simulink model "CF009A_GmOvrlStMgr"  (R2013b)
settings: Solver=FixedStepDiscrete  SolverMode=SingleTasking  StartTime=0.0  StopTime=1  FixedStep=0.002  RelTol=1e-3
values from neighbouring files (symbols this model uses):
  APASTACTV_CNT_U08 = DataDict.Constant    [CF009A_GmOvrlStMgr_DataDict.m]
  APASTCTRLAVL_CNT_U08 = DataDict.Constant    [CF009A_GmOvrlStMgr_DataDict.m]
  ARCHGLBPRM_2MILLISEC_SEC_F32 = DataDict.Constant    [CF009A_GmOvrlStMgr_DataDict.m]
  GmOvrlStMgrApaHwTqThd = DataDict.Calibration    [CF009A_GmOvrlStMgr_DataDict.m]
  GmOvrlStMgrApaHwTqTiThd = DataDict.Calibration    [CF009A_GmOvrlStMgr_DataDict.m]
  GmOvrlStMgrApaMfgEna = DataDict.Calibration    [CF009A_GmOvrlStMgr_DataDict.m]
  GmOvrlStMgrEscMfgEna = DataDict.Calibration    [CF009A_GmOvrlStMgr_DataDict.m]
  GmOvrlStMgrHaptcAmp = DataDict.Calibration    [CF009A_GmOvrlStMgr_DataDict.m]
  GmOvrlStMgrHaptcDurn = DataDict.Calibration    [CF009A_GmOvrlStMgr_DataDict.m]
  GmOvrlStMgrHaptcFrq = DataDict.Calibration    [CF009A_GmOvrlStMgr_DataDict.m]
  GmOvrlStMgrHaptcReactnTi = DataDict.Calibration    [CF009A_GmOvrlStMgr_DataDict.m]
  GmOvrlStMgrHaptcReqTiThd = DataDict.Calibration    [CF009A_GmOvrlStMgr_DataDict.m]
  GmOvrlStMgrHwAgTarLimr = DataDict.Calibration    [CF009A_GmOvrlStMgr_DataDict.m]
  GmOvrlStMgrLkaHwTqThd1 = DataDict.Calibration    [CF009A_GmOvrlStMgr_DataDict.m]
  GmOvrlStMgrLkaHwTqThd2 = DataDict.Calibration    [CF009A_GmOvrlStMgr_DataDict.m]
  GmOvrlStMgrLkaHwTqTiThd1 = DataDict.Calibration    [CF009A_GmOvrlStMgr_DataDict.m]
  GmOvrlStMgrLkaHwTqTiThd2 = DataDict.Calibration    [CF009A_GmOvrlStMgr_DataDict.m]
  GmOvrlStMgrLkaMfgEna = DataDict.Calibration    [CF009A_GmOvrlStMgr_DataDict.m]
  GmOvrlStMgrLoaMtgtnHaptcFbOffTi = DataDict.Calibration    [CF009A_GmOvrlStMgr_DataDict.m]
  GmOvrlStMgrLoaMtgtnHaptcFbOnTi = DataDict.Calibration    [CF009A_GmOvrlStMgr_DataDict.m]
  GmOvrlStMgrLoaMtgtnHaptcFbStrtOnTi = DataDict.Calibration    [CF009A_GmOvrlStMgr_DataDict.m]
  GmOvrlStMgrLoaMtgtnHaptcFbTqMax = DataDict.Calibration    [CF009A_GmOvrlStMgr_DataDict.m]
  GmOvrlStMgrLoaMtgtnHaptcFbTqMin = DataDict.Calibration    [CF009A_GmOvrlStMgr_DataDict.m]
  GmOvrlStMgrLoaMtgtnHaptcFbVehSpdMax = DataDict.Calibration    [CF009A_GmOvrlStMgr_DataDict.m]
  GmOvrlStMgrLoaMtgtnHaptcFbVehSpdMin = DataDict.Calibration    [CF009A_GmOvrlStMgr_DataDict.m]
  GmOvrlStMgrLoaMtgtnHaptcFrq = DataDict.Calibration    [CF009A_GmOvrlStMgr_DataDict.m]
  GmOvrlStMgrLoaMtgtnStrtHaptcAmp = DataDict.Calibration    [CF009A_GmOvrlStMgr_DataDict.m]
  GmOvrlStMgrLoaStIgnCntrThd = DataDict.Calibration    [CF009A_GmOvrlStMgr_DataDict.m]
  GmOvrlStMgrShiftLvrTiThd = DataDict.Calibration    [CF009A_GmOvrlStMgr_DataDict.m]
  GmOvrlStMgrStandStillThd = DataDict.Calibration    [CF009A_GmOvrlStMgr_DataDict.m]
  GmOvrlStMgrStandStillTiThd = DataDict.Calibration    [CF009A_GmOvrlStMgr_DataDict.m]
  HAPTCSTACTV_CNT_U08 = DataDict.Constant    [CF009A_GmOvrlStMgr_DataDict.m]
  HAPTCSTWAIT_CNT_U08 = DataDict.Constant    [CF009A_GmOvrlStMgr_DataDict.m]
  HWOSCNFRQMIN_HZ_F32 = DataDict.Constant    [CF009A_GmOvrlStMgr_DataDict.m]
  LKAFLTCNTRTHD_CNT_U08 = DataDict.Constant    [CF009A_GmOvrlStMgr_DataDict.m]
  LKAFLTTMRTHD_MILLISEC_U32 = DataDict.Constant    [CF009A_GmOvrlStMgr_DataDict.m]
  LKASTPRMNTFAILD_CNT_U08 = DataDict.Constant    [CF009A_GmOvrlStMgr_DataDict.m]
  LoaMtgtnThdExcdd = DataDict.NTC    [CF009A_GmOvrlStMgr_DataDict.m]
  MILLISECTO100MICROSECCNVN_CNT_U32 = DataDict.Constant    [CF009A_GmOvrlStMgr_DataDict.m]
  NODEBSTEP_CNT_U16 = DataDict.Constant    [CF009A_GmOvrlStMgr_DataDict.m]
undefined symbols (not defined in the file or in its folder): LoaSt1, NtcSts1, NVM_RequestResultType, SysSt1
libraries: simulink x13, Fil x6, NxtrNvM x4, NxtrLim x4, NxtrAbslt x3, NxtrSign x2, FixdToFloat x1, FloatToFixd x1, LnrIntrpn x1
(part 5 of 8)

== system CF009A_GmOvrlStMgr/GmOvrlStMgr/GmOvrlStMgrPer1/ApaIntv/Timer for ApaIntv/If Action Subsystem2 ==
  Action Port : ActionPort  ActionType=elseif
  CopyRight2 : Subsystem  Description=|  mask(Copyright Information){none=on}
      | Copyright info block.                                               
      |                                                                     
      | Place copyright information at the top of every subsystem in design.
      mask prompts: none "No parameters"
      mask help: Place copyright information at the top of every subsystem in design.
      mask Display:
      | NxtrConf = 'Nexteer Confidential';
      | 
      | sys = bdroot; %handle for the current model ("system")
      | first = get_param(sys,'Created');
      | first = first(end-3:end);  %year is last four digits
      | 
      | last = get_param(sys,'LastModifiedDate');
      | if isempty(last)
      |     last = datestr(now,'yyyy');
      | else
      |     last = last(end-3:end);
      | end
      | 
      | if strcmp(first,last)
      |     fprintf('%s -- Copyright %s Nexteer',NxtrConf,first)
      | else
      |     fprintf('%s -- %s%s- %s Nexteer',NxtrConf,char(169),first,last)
      | end
  Data Store Read : DataStoreRead  DataStoreName=PrevApaIntvRefTi
  GetTiSpan100MicroSec32bit1 : Subsystem
  Out1 : Outport
  wires:
  GetTiSpan100MicroSec32bit1/1(TiSpan) -> Out1/1
  Data Store Read/1 -> GetTiSpan100MicroSec32bit1/1(RefTmr)

== system CF009A_GmOvrlStMgr/GmOvrlStMgr/GmOvrlStMgrPer1/HaptcStTransActvToWaitFlg/ElpseTi/CopyRight2 ==

== system CF009A_GmOvrlStMgr/GmOvrlStMgr/GmOvrlStMgrPer1/HaptcStTransActvToWaitFlg/ElpseTi/GetTiSpan100MicroSec32bit ==
  note: Subtract original reference time
  note: seconds
  note: microseconds
  note: counts
  note: Wrap-to-zero
  note: 1 count = 100 uSec
  note: Get current system time
  note: GetTiSpan100MicroSec32bit
  note: Created Aug 18, 2015
      | Modified Oct 21, 2015
      | Modified Oct 30, 2015
      | Kevin Derry
  RefTmr : Inport
  CopyRight2 : Subsystem  Description=|  mask(Copyright Information){none=on}
      | Copyright info block.                                               
      |                                                                     
      | Place copyright information at the top of every subsystem in design.
      mask prompts: none "No parameters"
      mask help: Place copyright information at the top of every subsystem in design.
      mask Display:
      | NxtrConf = 'Nexteer Confidential';
      | 
      | sys = bdroot; %handle for the current model ("system")
      | first = get_param(sys,'Created');
      | if(isempty(first))
      |     first = datestr(now,'yyyy');
      | else
      |     first = first(end-3:end);  %year is last four digits
      | end
      | 
      | last = get_param(sys,'LastModifiedDate');
      | if isempty(last)
      |     last = datestr(now,'yyyy');
      | else
      |     last = last(end-3:end);
      | end
      | 
      | if strcmp(first,last)
      |     fprintf('%s -- Copyright %s Nexteer',NxtrConf,first)
      | else
      |     fprintf('%s -- %s%s- %s Nexteer',NxtrConf,char(169),first,last)
      | end
  Count per uSec : Constant  Value=0.01
  Data Store Read1 : DataStoreRead  DataStoreName=SimnTi
  Data Type Conversion2 : DataTypeConversion  OutDataTypeStr=uint32
  Divide1 : Product  Inputs=**
  Divide2 : Product  Inputs=*/
  If : If  NumInputs=2  IfExpression=u1 >= u2
  Max Counts : Constant  Value=2^32-1
  Merge : Merge
  No wrapping : Subsystem  TreatAsAtomicUnit=on
  Product2 : Product
  Product3 : Product
  Rounding : Rounding
  Subtract3 : Sum  Inputs=+-
  Wrapping : Subsystem  TreatAsAtomicUnit=on
  uSec per Sec : Constant  Value=1000000
  TiSpan : Outport
  wires:
  Wrapping/1(Out1) -> Merge/2
  No wrapping/1(Out1) -> Merge/1
  If/2 -> Wrapping/Action
  If/1 -> No wrapping/Action
  Product3/1 -> Subtract3/2
  Subtract3/1 -> Data Type Conversion2/1
  Rounding/1 -> Product3/1
  Divide2/1 -> Rounding/1
  Max Counts/1 -> Divide2/2, Product3/2
  Divide1/1 -> Divide2/1, Subtract3/1
  Product2/1 -> Divide1/1
  Data Store Read1/1 -> Product2/1
  Count per uSec/1 -> Divide1/2
  uSec per Sec/1 -> Product2/2
  Merge/1 -> TiSpan/1
  RefTmr/1 -> If/2, No wrapping/2(ref), Wrapping/2(ref)
  Data Type Conversion2/1 -> If/1, No wrapping/1(new), Wrapping/1(new)

== system CF009A_GmOvrlStMgr/GmOvrlStMgr/GmOvrlStMgrPer1/HaptcStTransActvToWaitFlg/ElpseTi/Set False Subsystem ==
  Action Port : ActionPort  ActionType=else
  Constant1 : Constant  RequirementInfo={} %GIDa_7a5b8ee3_9c22_45c3_98e2_7098368aea92  Value=false  OutDataTypeStr=boolean
      settings: AttributesFormatString=%<OutDataTypeStr>
  CopyRight2 : Subsystem  Description=|  mask(Copyright Information){none=on}
      | Copyright info block.                                               
      |                                                                     
      | Place copyright information at the top of every subsystem in design.
      mask prompts: none "No parameters"
      mask help: Place copyright information at the top of every subsystem in design.
      mask Display:
      | NxtrConf = 'Nexteer Confidential';
      | 
      | sys = bdroot; %handle for the current model ("system")
      | first = get_param(sys,'Created');
      | first = first(end-3:end);  %year is last four digits
      | 
      | last = get_param(sys,'LastModifiedDate');
      | if isempty(last)
      |     last = datestr(now,'yyyy');
      | else
      |     last = last(end-3:end);
      | end
      | 
      | if strcmp(first,last)
      |     fprintf('%s -- Copyright %s Nexteer',NxtrConf,first)
      | else
      |     fprintf('%s -- %s%s- %s Nexteer',NxtrConf,char(169),first,last)
      | end
  Out1 : Outport
  wires:
  Constant1/1 -> Out1/1

== system CF009A_GmOvrlStMgr/GmOvrlStMgr/GmOvrlStMgrPer1/HaptcStTransActvToWaitFlg/ElpseTi/Set True Subsystem ==
  Action Port : ActionPort  ActionType=then
  Constant13 : Constant  RequirementInfo={} %GIDa_d2a44b6e_d583_493a_9335_9403f2dad45d  Value=true  OutDataTypeStr=boolean
      settings: AttributesFormatString=%<OutDataTypeStr>
  CopyRight2 : Subsystem  Description=|  mask(Copyright Information){none=on}
      | Copyright info block.                                               
      |                                                                     
      | Place copyright information at the top of every subsystem in design.
      mask prompts: none "No parameters"
      mask help: Place copyright information at the top of every subsystem in design.
      mask Display:
      | NxtrConf = 'Nexteer Confidential';
      | 
      | sys = bdroot; %handle for the current model ("system")
      | first = get_param(sys,'Created');
      | first = first(end-3:end);  %year is last four digits
      | 
      | last = get_param(sys,'LastModifiedDate');
      | if isempty(last)
      |     last = datestr(now,'yyyy');
      | else
      |     last = last(end-3:end);
      | end
      | 
      | if strcmp(first,last)
      |     fprintf('%s -- Copyright %s Nexteer',NxtrConf,first)
      | else
      |     fprintf('%s -- %s%s- %s Nexteer',NxtrConf,char(169),first,last)
      | end
  Out1 : Outport
  wires:
  Constant13/1 -> Out1/1

== system CF009A_GmOvrlStMgr/GmOvrlStMgr/GmOvrlStMgrPer1/HaptcStTransActvToWaitFlg/RefTi/CopyRight2 ==

== system CF009A_GmOvrlStMgr/GmOvrlStMgr/GmOvrlStMgrPer1/HaptcStTransActvToWaitFlg/RefTi/GetRefTmr100MicroSec32bit ==
  note: 1 count = 100 uSec
  note: seconds
  note: microseconds
  note: counts
  note: Wrap-to-zero
  note: GetRefTmr100MicroSec32bit
  note: Created Aug 18, 2015
      | Modified Oct 21, 2015
      | Modified Oct 30, 2015
      | Kevin Derry
  CopyRight2 : Subsystem  Description=|  mask(Copyright Information){none=on}
      | Copyright info block.                                               
      |                                                                     
      | Place copyright information at the top of every subsystem in design.
      mask prompts: none "No parameters"
      mask help: Place copyright information at the top of every subsystem in design.
      mask Display:
      | NxtrConf = 'Nexteer Confidential';
      | 
      | sys = bdroot; %handle for the current model ("system")
      | first = get_param(sys,'Created');
      | if(isempty(first))
      |     first = datestr(now,'yyyy');
      | else
      |     first = first(end-3:end);  %year is last four digits
      | end
      | 
      | last = get_param(sys,'LastModifiedDate');
      | if isempty(last)
      |     last = datestr(now,'yyyy');
      | else
      |     last = last(end-3:end);
      | end
      | 
      | if strcmp(first,last)
      |     fprintf('%s -- Copyright %s Nexteer',NxtrConf,first)
      | else
      |     fprintf('%s -- %s%s- %s Nexteer',NxtrConf,char(169),first,last)
      | end
  Count per uSec : Constant  Value=0.01
  Data Store Read1 : DataStoreRead  DataStoreName=SimnTi
  Data Type Conversion1 : DataTypeConversion  OutDataTypeStr=uint32
  Divide1 : Product  Inputs=**
  Divide2 : Product  Inputs=*/
  Max Counts : Constant  Value=2^32-1
  Product1 : Product
  Product2 : Product
  Rounding : Rounding
  Subtract1 : Sum  Inputs=+-
  uSec per Sec : Constant  Value=1000000
  RefTmr : Outport
  wires:
  Product2/1 -> Subtract1/2
  Subtract1/1 -> Data Type Conversion1/1
  Rounding/1 -> Product2/1
  Divide2/1 -> Rounding/1
  Max Counts/1 -> Divide2/2, Product2/2
  Divide1/1 -> Divide2/1, Subtract1/1
  Product1/1 -> Divide1/1
  Count per uSec/1 -> Divide1/2
  uSec per Sec/1 -> Product1/2
  Data Type Conversion1/1 -> RefTmr/1
  Data Store Read1/1 -> Product1/1

== system CF009A_GmOvrlStMgr/GmOvrlStMgr/GmOvrlStMgrPer1/HwAgServo/If Action Subsystem/ApaStatusActive ==
  note: Code uses magic number
  Action Port : ActionPort  ActionType=then
  Constant : Constant  Value=false
  Constant1 : Constant  Value=0  OutDataTypeStr=single
  CopyRight2 : Subsystem  Description=|  mask(Copyright Information){none=on}
      | Copyright info block.                                               
      |                                                                     
      | Place copyright information at the top of every subsystem in design.
      mask prompts: none "No parameters"
      mask help: Place copyright information at the top of every subsystem in design.
      mask Display:
      | NxtrConf = 'Nexteer Confidential';
      | 
      | sys = bdroot; %handle for the current model ("system")
      | first = get_param(sys,'Created');
      | if(isempty(first))
      |     first = datestr(now,'yyyy');
      | else
      |     first = first(end-3:end);  %year is last four digits
      | end
      | 
      | last = get_param(sys,'LastModifiedDate');
      | if isempty(last)
      |     last = datestr(now,'yyyy');
      | else
      |     last = last(end-3:end);
      | end
      | 
      | if strcmp(first,last)
      |     fprintf('%s -- Copyright %s Nexteer',NxtrConf,first)
      | else
      |     fprintf('%s -- %s%s- %s Nexteer',NxtrConf,char(169),first,last)
      | end
  HwAgServoEna : Outport
  HwAgServoCmd : Outport  Port=2
  wires:
  Constant/1 -> HwAgServoEna/1
  Constant1/1 -> HwAgServoCmd/1

== system CF009A_GmOvrlStMgr/GmOvrlStMgr/GmOvrlStMgrPer1/HwAgServo/If Action Subsystem/ApaStatusNotActive ==
  HwAgTraj : Inport
  Action Port : ActionPort  ActionType=else
  Constant : Constant  Value=true
  CopyRight2 : Subsystem  Description=|  mask(Copyright Information){none=on}
      | Copyright info block.                                               
      |                                                                     
      | Place copyright information at the top of every subsystem in design.
      mask prompts: none "No parameters"
      mask help: Place copyright information at the top of every subsystem in design.
      mask Display:
      | NxtrConf = 'Nexteer Confidential';
      | 
      | sys = bdroot; %handle for the current model ("system")
      | first = get_param(sys,'Created');
      | if(isempty(first))
      |     first = datestr(now,'yyyy');
      | else
      |     first = first(end-3:end);  %year is last four digits
      | end
      | 
      | last = get_param(sys,'LastModifiedDate');
      | if isempty(last)
      |     last = datestr(now,'yyyy');
      | else
      |     last = last(end-3:end);
      | end
      | 
      | if strcmp(first,last)
      |     fprintf('%s -- Copyright %s Nexteer',NxtrConf,first)
      | else
      |     fprintf('%s -- %s%s- %s Nexteer',NxtrConf,char(169),first,last)
      | end
  HwAgServoCmd : Outport
  HwAgServoEna : Outport  Port=2
  wires:
  Constant/1 -> HwAgServoEna/1
  HwAgTraj/1 -> HwAgServoCmd/1

== system CF009A_GmOvrlStMgr/GmOvrlStMgr/GmOvrlStMgrPer1/HwAgServo/If Action Subsystem/CopyRight2 ==

== system CF009A_GmOvrlStMgr/GmOvrlStMgr/GmOvrlStMgrPer1/HwAgServo/If Action Subsystem1/ApaStatusActive ==
  HwAgTarLimd : Inport
  Action Port : ActionPort  ActionType=then
  Constant : Constant  Value=true
  CopyRight2 : Subsystem  Description=|  mask(Copyright Information){none=on}
      | Copyright info block.                                               
      |                                                                     
      | Place copyright information at the top of every subsystem in design.
      mask prompts: none "No parameters"
      mask help: Place copyright information at the top of every subsystem in design.
      mask Display:
      | NxtrConf = 'Nexteer Confidential';
      | 
      | sys = bdroot; %handle for the current model ("system")
      | first = get_param(sys,'Created');
      | if(isempty(first))
      |     first = datestr(now,'yyyy');
      | else
      |     first = first(end-3:end);  %year is last four digits
      | end
      | 
      | last = get_param(sys,'LastModifiedDate');
      | if isempty(last)
      |     last = datestr(now,'yyyy');
      | else
      |     last = last(end-3:end);
      | end
      | 
      | if strcmp(first,last)
      |     fprintf('%s -- Copyright %s Nexteer',NxtrConf,first)
      | else
      |     fprintf('%s -- %s%s- %s Nexteer',NxtrConf,char(169),first,last)
      | end
  HwAgServoCmd : Outport
  HwAgServoEna : Outport  Port=2
  wires:
  Constant/1 -> HwAgServoEna/1
  HwAgTarLimd/1 -> HwAgServoCmd/1

== system CF009A_GmOvrlStMgr/GmOvrlStMgr/GmOvrlStMgrPer1/HwAgServo/If Action Subsystem1/ApaStatusNotActive ==
  note: Code uses magic number
  Action Port : ActionPort  ActionType=else
  Constant1 : Constant  Value=false
  Constant2 : Constant  Value=0  OutDataTypeStr=single
  CopyRight2 : Subsystem  Description=|  mask(Copyright Information){none=on}
      | Copyright info block.                                               
      |                                                                     
      | Place copyright information at the top of every subsystem in design.
      mask prompts: none "No parameters"
      mask help: Place copyright information at the top of every subsystem in design.
      mask Display:
      | NxtrConf = 'Nexteer Confidential';
      | 
      | sys = bdroot; %handle for the current model ("system")
      | first = get_param(sys,'Created');
      | if(isempty(first))
      |     first = datestr(now,'yyyy');
      | else
      |     first = first(end-3:end);  %year is last four digits
      | end
      | 
      | last = get_param(sys,'LastModifiedDate');
      | if isempty(last)
      |     last = datestr(now,'yyyy');
      | else
      |     last = last(end-3:end);
      | end
      | 
      | if strcmp(first,last)
      |     fprintf('%s -- Copyright %s Nexteer',NxtrConf,first)
      | else
      |     fprintf('%s -- %s%s- %s Nexteer',NxtrConf,char(169),first,last)
      | end
  HwAgServoEna : Outport
  HwAgServoCmd : Outport  Port=2
  wires:
  Constant1/1 -> HwAgServoEna/1
  Constant2/1 -> HwAgServoCmd/1

== system CF009A_GmOvrlStMgr/GmOvrlStMgr/GmOvrlStMgrPer1/HwAgServo/If Action Subsystem1/CopyRight2 ==

== system CF009A_GmOvrlStMgr/GmOvrlStMgr/GmOvrlStMgrPer1/Inct_IgnCntr_Once/IgnCntr/CopyRight2 ==

== system CF009A_GmOvrlStMgr/GmOvrlStMgr/GmOvrlStMgrPer1/LKAIntv/HwTqLkaTqSignEqu/CopyRight2 ==

== system CF009A_GmOvrlStMgr/GmOvrlStMgr/GmOvrlStMgrPer1/LKAIntv/HwTqLkaTqSignEqu/GetRefTmr100MicroSec32bit ==
  note: Created Aug 18, 2015
      | Modified Oct 21, 2015
      | Modified Oct 30, 2015
      | Kevin Derry
  note: GetRefTmr100MicroSec32bit
  note: Wrap-to-zero
  note: counts
  note: microseconds
  note: seconds
  note: 1 count = 100 uSec
  CopyRight2 : Subsystem  Description=|  mask(Copyright Information){none=on}
      | Copyright info block.                                               
      |                                                                     
      | Place copyright information at the top of every subsystem in design.
      mask prompts: none "No parameters"
      mask help: Place copyright information at the top of every subsystem in design.
      mask Display:
      | NxtrConf = 'Nexteer Confidential';
      | 
      | sys = bdroot; %handle for the current model ("system")
      | first = get_param(sys,'Created');
      | if(isempty(first))
      |     first = datestr(now,'yyyy');
      | else
      |     first = first(end-3:end);  %year is last four digits
      | end
      | 
      | last = get_param(sys,'LastModifiedDate');
      | if isempty(last)
      |     last = datestr(now,'yyyy');
      | else
      |     last = last(end-3:end);
      | end
      | 
      | if strcmp(first,last)
      |     fprintf('%s -- Copyright %s Nexteer',NxtrConf,first)
      | else
      |     fprintf('%s -- %s%s- %s Nexteer',NxtrConf,char(169),first,last)
      | end
  Count per uSec : Constant  Value=0.01
  Data Store Read1 : DataStoreRead  DataStoreName=SimnTi
  Data Type Conversion1 : DataTypeConversion  OutDataTypeStr=uint32
  Divide1 : Product  Inputs=**
  Divide2 : Product  Inputs=*/
  Max Counts : Constant  Value=2^32-1
  Product1 : Product
  Product2 : Product
  Rounding : Rounding
  Subtract1 : Sum  Inputs=+-
  uSec per Sec : Constant  Value=1000000
  RefTmr : Outport
  wires:
  Data Store Read1/1 -> Product1/1
  Data Type Conversion1/1 -> RefTmr/1
  uSec per Sec/1 -> Product1/2
  Count per uSec/1 -> Divide1/2
  Product1/1 -> Divide1/1
  Divide1/1 -> Subtract1/1, Divide2/1
  Max Counts/1 -> Product2/2, Divide2/2
  Divide2/1 -> Rounding/1
  Rounding/1 -> Product2/1
  Subtract1/1 -> Data Type Conversion1/1
  Product2/1 -> Subtract1/2

== system CF009A_GmOvrlStMgr/GmOvrlStMgr/GmOvrlStMgrPer1/LKAIntv/HwTqLkaTqSignEqu/GetRefTmr100MicroSec32bit_1 ==
  note: 1 count = 100 uSec
  note: seconds
  note: microseconds
  note: counts
  note: Wrap-to-zero
  note: GetRefTmr100MicroSec32bit
  note: Created Aug 18, 2015
      | Modified Oct 21, 2015
      | Modified Oct 30, 2015
      | Kevin Derry
  CopyRight2 : Subsystem  Description=|  mask(Copyright Information){none=on}
      | Copyright info block.                                               
      |                                                                     
      | Place copyright information at the top of every subsystem in design.
      mask prompts: none "No parameters"
      mask help: Place copyright information at the top of every subsystem in design.
      mask Display:
      | NxtrConf = 'Nexteer Confidential';
      | 
      | sys = bdroot; %handle for the current model ("system")
      | first = get_param(sys,'Created');
      | if(isempty(first))
      |     first = datestr(now,'yyyy');
      | else
      |     first = first(end-3:end);  %year is last four digits
      | end
      | 
      | last = get_param(sys,'LastModifiedDate');
      | if isempty(last)
      |     last = datestr(now,'yyyy');
      | else
      |     last = last(end-3:end);
      | end
      | 
      | if strcmp(first,last)
      |     fprintf('%s -- Copyright %s Nexteer',NxtrConf,first)
      | else
      |     fprintf('%s -- %s%s- %s Nexteer',NxtrConf,char(169),first,last)
      | end
  Count per uSec : Constant  Value=0.01
  Data Store Read1 : DataStoreRead  DataStoreName=SimnTi
  Data Type Conversion1 : DataTypeConversion  OutDataTypeStr=uint32
  Divide1 : Product  Inputs=**
  Divide2 : Product  Inputs=*/
  Max Counts : Constant  Value=2^32-1
  Product1 : Product
  Product2 : Product
  Rounding : Rounding
  Subtract1 : Sum  Inputs=+-
  uSec per Sec : Constant  Value=1000000
  RefTmr : Outport
  wires:
  Product2/1 -> Subtract1/2
  Subtract1/1 -> Data Type Conversion1/1
  Rounding/1 -> Product2/1
  Divide2/1 -> Rounding/1
  Max Counts/1 -> Divide2/2, Product2/2
  Divide1/1 -> Divide2/1, Subtract1/1
  Product1/1 -> Divide1/1
  Count per uSec/1 -> Divide1/2
  uSec per Sec/1 -> Product1/2
  Data Type Conversion1/1 -> RefTmr/1
  Data Store Read1/1 -> Product1/1

== system CF009A_GmOvrlStMgr/GmOvrlStMgr/GmOvrlStMgrPer1/LKAIntv/HwTqLkaTqSignNotEqu/ChkTmr1 ==
  Action Port : ActionPort  ActionType=then
  Constant : Constant  RequirementInfo={} %GIDa_31957342_5e2f_4bc5_989e_9132f947ba0e  Value=GmOvrlStMgrLkaHwTqTiThd1
  Constant1 : Constant  Value=MILLISECTO100MICROSECCNVN_CNT_U32
  CopyRight2 : Subsystem  Description=|  mask(Copyright Information){none=on}
      | Copyright info block.                                               
      |                                                                     
      | Place copyright information at the top of every subsystem in design.
      mask prompts: none "No parameters"
      mask help: Place copyright information at the top of every subsystem in design.
      mask Display:
      | NxtrConf = 'Nexteer Confidential';
      | 
      | sys = bdroot; %handle for the current model ("system")
      | first = get_param(sys,'Created');
      | if(isempty(first))
      |     first = datestr(now,'yyyy');
      | else
      |     first = first(end-3:end);  %year is last four digits
      | end
      | 
      | last = get_param(sys,'LastModifiedDate');
      | if isempty(last)
      |     last = datestr(now,'yyyy');
      | else
      |     last = last(end-3:end);
      | end
      | 
      | if strcmp(first,last)
      |     fprintf('%s -- Copyright %s Nexteer',NxtrConf,first)
      | else
      |     fprintf('%s -- %s%s- %s Nexteer',NxtrConf,char(169),first,last)
      | end
  Data Store Read : DataStoreRead  DataStoreName=LkaIntvRefTi1
  Data Store Write1 : DataStoreWrite  DataStoreName=LkaIntvRefTi2
  GetRefTmr100MicroSec32bit : Subsystem
  GetTiSpan100MicroSec32bit : Subsystem
  If1 : If  IfExpression=u1
  LKAIntvTi1Elpd : Subsystem
  LKAIntvTi1NotElpd : Subsystem
  Merge3 : Merge
  Product1 : Product
  Relational Operator : RelationalOperator  OutDataTypeStr=boolean
  Out1 : Outport
  wires:
  Merge3/1 -> Out1/1
  LKAIntvTi1NotElpd/1(Out1) -> Merge3/2
  LKAIntvTi1Elpd/1(Out1) -> Merge3/1
  If1/2 -> LKAIntvTi1NotElpd/Action
  If1/1 -> LKAIntvTi1Elpd/Action
  Constant/1 -> Product1/1
  Product1/1 -> Relational Operator/2
  Constant1/1 -> Product1/2
  Relational Operator/1 -> If1/1
  GetTiSpan100MicroSec32bit/1(TiSpan) -> Relational Operator/1
  Data Store Read/1 -> GetTiSpan100MicroSec32bit/1(RefTmr)
  GetRefTmr100MicroSec32bit/1(RefTmr) -> Data Store Write1/1

== system CF009A_GmOvrlStMgr/GmOvrlStMgr/GmOvrlStMgrPer1/LKAIntv/HwTqLkaTqSignNotEqu/ChkTmr2 ==
  Action Port : ActionPort  ActionType=elseif
  Constant : Constant  RequirementInfo={} %GIDa_932db252_e6c8_4b41_be46_d3f1492e3714  Value=GmOvrlStMgrLkaHwTqTiThd2
  Constant1 : Constant  Value=MILLISECTO100MICROSECCNVN_CNT_U32
  CopyRight2 : Subsystem  Description=|  mask(Copyright Information){none=on}
      | Copyright info block.                                               
      |                                                                     
      | Place copyright information at the top of every subsystem in design.
      mask prompts: none "No parameters"
      mask help: Place copyright information at the top of every subsystem in design.
      mask Display:
      | NxtrConf = 'Nexteer Confidential';
      | 
      | sys = bdroot; %handle for the current model ("system")
      | first = get_param(sys,'Created');
      | first = first(end-3:end);  %year is last four digits
      | 
      | last = get_param(sys,'LastModifiedDate');
      | if isempty(last)
      |     last = datestr(now,'yyyy');
      | else
      |     last = last(end-3:end);
      | end
      | 
      | if strcmp(first,last)
      |     fprintf('%s -- Copyright %s Nexteer',NxtrConf,first)
      | else
      |     fprintf('%s -- %s%s- %s Nexteer',NxtrConf,char(169),first,last)
      | end
  Data Store Read : DataStoreRead  DataStoreName=LkaIntvRefTi2
  Data Store Write9 : DataStoreWrite  DataStoreName=LkaIntvRefTi1
  GetRefTmr100MicroSec32bit : Subsystem
  GetTiSpan100MicroSec32bit : Subsystem
  If1 : If  IfExpression=u1
  LKAIntvTi2Elpd : Subsystem
  LKAIntvTi2NotElpd : Subsystem
  Merge3 : Merge
  Product1 : Product
  Relational Operator : RelationalOperator  OutDataTypeStr=boolean
  Out1 : Outport
  wires:
  Data Store Read/1 -> GetTiSpan100MicroSec32bit/1(RefTmr)
  GetTiSpan100MicroSec32bit/1(TiSpan) -> Relational Operator/1
  Relational Operator/1 -> If1/1
  Constant1/1 -> Product1/2
  Product1/1 -> Relational Operator/2
  Constant/1 -> Product1/1
  If1/1 -> LKAIntvTi2Elpd/Action
  If1/2 -> LKAIntvTi2NotElpd/Action
  LKAIntvTi2NotElpd/1(Out1) -> Merge3/2
  Merge3/1 -> Out1/1
  GetRefTmr100MicroSec32bit/1(RefTmr) -> Data Store Write9/1
  LKAIntvTi2Elpd/1(Out1) -> Merge3/1

== system CF009A_GmOvrlStMgr/GmOvrlStMgr/GmOvrlStMgrPer1/LKAIntv/HwTqLkaTqSignNotEqu/CopyRight2 ==

== system CF009A_GmOvrlStMgr/GmOvrlStMgr/GmOvrlStMgrPer1/LKAIntv/HwTqLkaTqSignNotEqu/TmrRst ==
  Action Port : ActionPort  ActionType=else
  Constant13 : Constant  RequirementInfo={} %GIDa_6df395ac_9b22_44c0_88b8_346f6118ff67  Value=false  OutDataTypeStr=boolean
      settings: AttributesFormatString=%<OutDataTypeStr>
  CopyRight2 : Subsystem  Description=|  mask(Copyright Information){none=on}
      | Copyright info block.                                               
      |                                                                     
      | Place copyright information at the top of every subsystem in design.
      mask prompts: none "No parameters"
      mask help: Place copyright information at the top of every subsystem in design.
      mask Display:
      | NxtrConf = 'Nexteer Confidential';
      | 
      | sys = bdroot; %handle for the current model ("system")
      | first = get_param(sys,'Created');
      | first = first(end-3:end);  %year is last four digits
      | 
      | last = get_param(sys,'LastModifiedDate');
      | if isempty(last)
      |     last = datestr(now,'yyyy');
      | else
      |     last = last(end-3:end);
      | end
      | 
      | if strcmp(first,last)
      |     fprintf('%s -- Copyright %s Nexteer',NxtrConf,first)
      | else
      |     fprintf('%s -- %s%s- %s Nexteer',NxtrConf,char(169),first,last)
      | end
  Data Store Write1 : DataStoreWrite  DataStoreName=LkaIntvRefTi2
  Data Store Write9 : DataStoreWrite  DataStoreName=LkaIntvRefTi1
  GetRefTmr100MicroSec32bit : Subsystem
  GetRefTmr100MicroSec32bit_1 : Subsystem
  Out1 : Outport
  wires:
  Constant13/1 -> Out1/1
  GetRefTmr100MicroSec32bit/1(RefTmr) -> Data Store Write9/1
  GetRefTmr100MicroSec32bit_1/1(RefTmr) -> Data Store Write1/1

== system CF009A_GmOvrlStMgr/GmOvrlStMgr/GmOvrlStMgrPer1/LkaCheck/ProcessInp/CopyRight2 ==

== system CF009A_GmOvrlStMgr/GmOvrlStMgr/GmOvrlStMgrPer1/LkaCheck/ProcessInp/Inct_LkaFltCntr_One ==
  Action Port : ActionPort  ActionType=then
  Constant1 : Constant  Value=LKAFLTCNTRTHD_CNT_U08
  Constant2 : Constant  Value=LKAFLTCNTRTHD_CNT_U08
  CopyRight2 : Subsystem  Description=|  mask(Copyright Information){none=on}
      | Copyright info block.                                               
      |                                                                     
      | Place copyright information at the top of every subsystem in design.
      mask prompts: none "No parameters"
      mask help: Place copyright information at the top of every subsystem in design.
      mask Display:
      | NxtrConf = 'Nexteer Confidential';
      | 
      | sys = bdroot; %handle for the current model ("system")
      | first = get_param(sys,'Created');
      | if(isempty(first))
      |     first = datestr(now,'yyyy');
      | else
      |     first = first(end-3:end);  %year is last four digits
      | end
      | 
      | last = get_param(sys,'LastModifiedDate');
      | if isempty(last)
      |     last = datestr(now,'yyyy');
      | else
      |     last = last(end-3:end);
      | end
      | 
      | if strcmp(first,last)
      |     fprintf('%s -- Copyright %s Nexteer',NxtrConf,first)
      | else
      |     fprintf('%s -- %s%s- %s Nexteer',NxtrConf,char(169),first,last)
      | end
  Data Store Read1 : DataStoreRead  DataStoreName=LkaFltCntr
  Data Store Read2 : DataStoreRead  DataStoreName=LkaFltCntr
  Data Store Write1 : DataStoreWrite  DataStoreName=LkaFltCntr
  If : If  IfExpression=u1
  Inct One : Subsystem  TreatAsAtomicUnit=on
  Merge : Merge
  Relational Operator : RelationalOperator  Operator=<  OutDataTypeStr=boolean
  Saturate At 255 : Subsystem  TreatAsAtomicUnit=on
  LkaFltCntr : Outport
  wires:
  Data Store Read1/1 -> Relational Operator/1
  Relational Operator/1 -> If/1
  If/1 -> Inct One/Action
  Data Store Read2/1 -> Inct One/1(In1)
  Inct One/1(Out1) -> Merge/1
  Merge/1 -> LkaFltCntr/1, Data Store Write1/1
  Saturate At 255/1(Out1) -> Merge/2
  If/2 -> Saturate At 255/Action
  Constant2/1 -> Saturate At 255/1(In1)
  Constant1/1 -> Relational Operator/2

== system CF009A_GmOvrlStMgr/GmOvrlStMgr/GmOvrlStMgrPer1/LkaCheck/SetDefVal/CopyRight2 ==

== system CF009A_GmOvrlStMgr/GmOvrlStMgr/GmOvrlStMgrPer1/LkaCheck/TmrElpdDetn/CopyRight2 ==

== system CF009A_GmOvrlStMgr/GmOvrlStMgr/GmOvrlStMgrPer1/LkaCheck/TmrElpdDetn/GetTiSpan100MicroSec32bit ==
  note: Subtract original reference time
  note: seconds
  note: microseconds
  note: counts
  note: Wrap-to-zero
  note: 1 count = 100 uSec
  note: Get current system time
  note: GetTiSpan100MicroSec32bit
  note: Created Aug 18, 2015
      | Modified Oct 21, 2015
      | Modified Oct 30, 2015
      | Kevin Derry
  RefTmr : Inport
  CopyRight2 : Subsystem  Description=|  mask(Copyright Information){none=on}
      | Copyright info block.                                               
      |                                                                     
      | Place copyright information at the top of every subsystem in design.
      mask prompts: none "No parameters"
      mask help: Place copyright information at the top of every subsystem in design.
      mask Display:
      | NxtrConf = 'Nexteer Confidential';
      | 
      | sys = bdroot; %handle for the current model ("system")
      | first = get_param(sys,'Created');
      | if(isempty(first))
      |     first = datestr(now,'yyyy');
      | else
      |     first = first(end-3:end);  %year is last four digits
      | end
      | 
      | last = get_param(sys,'LastModifiedDate');
      | if isempty(last)
      |     last = datestr(now,'yyyy');
      | else
      |     last = last(end-3:end);
      | end
      | 
      | if strcmp(first,last)
      |     fprintf('%s -- Copyright %s Nexteer',NxtrConf,first)
      | else
      |     fprintf('%s -- %s%s- %s Nexteer',NxtrConf,char(169),first,last)
      | end
  Count per uSec : Constant  Value=0.01
  Data Store Read1 : DataStoreRead  DataStoreName=SimnTi
  Data Type Conversion2 : DataTypeConversion  OutDataTypeStr=uint32
  Divide1 : Product  Inputs=**
  Divide2 : Product  Inputs=*/
  If : If  NumInputs=2  IfExpression=u1 >= u2
  Max Counts : Constant  Value=2^32-1
  Merge : Merge
  No wrapping : Subsystem  TreatAsAtomicUnit=on
  Product2 : Product
  Product3 : Product
  Rounding : Rounding
  Subtract3 : Sum  Inputs=+-
  Wrapping : Subsystem  TreatAsAtomicUnit=on
  uSec per Sec : Constant  Value=1000000
  TiSpan : Outport
  wires:
  Wrapping/1(Out1) -> Merge/2
  No wrapping/1(Out1) -> Merge/1
  If/2 -> Wrapping/Action
  If/1 -> No wrapping/Action
  Product3/1 -> Subtract3/2
  Subtract3/1 -> Data Type Conversion2/1
  Rounding/1 -> Product3/1
  Divide2/1 -> Rounding/1
  Max Counts/1 -> Divide2/2, Product3/2
  Divide1/1 -> Divide2/1, Subtract3/1
  Product2/1 -> Divide1/1
  Data Store Read1/1 -> Product2/1
  Count per uSec/1 -> Divide1/2
  uSec per Sec/1 -> Product2/2
  Merge/1 -> TiSpan/1
  RefTmr/1 -> If/2, No wrapping/2(ref), Wrapping/2(ref)
  Data Type Conversion2/1 -> If/1, No wrapping/1(new), Wrapping/1(new)

== system CF009A_GmOvrlStMgr/GmOvrlStMgr/GmOvrlStMgrPer1/LoaStLimdOrSwBasdMtgtn/Set_false_LoaStLimdOrSwBasdMtgtn/CopyRight2 ==

== system CF009A_GmOvrlStMgr/GmOvrlStMgr/GmOvrlStMgrPer1/LoaStLimdOrSwBasdMtgtn/Set_true_LoaStLimdOrSwBasdMtgtn/CopyRight2 ==

== system CF009A_GmOvrlStMgr/GmOvrlStMgr/GmOvrlStMgrPer1/SysStOperate/Chk_LoaSt_IgnCntr_ AtStartUp/CopyRight2 ==

== system CF009A_GmOvrlStMgr/GmOvrlStMgr/GmOvrlStMgrPer1/SysStOperate/Chk_LoaSt_IgnCntr_ AtStartUp/HaptcFbOn ==
  Action Port : ActionPort  ActionType=then
  Constant : Constant  RequirementInfo={} %GIDa_d634b896_4353_4d58_aab3_1388ff4e5a7e  Value=GmOvrlStMgrLoaMtgtnHaptcFbStrtOnTi
  Constant1 : Constant  Value=MILLISECTO100MICROSECCNVN_CNT_U32
  Constant13 : Constant  RequirementInfo={} %GIDa_262c0b0f_a1c7_4cb6_a322_56f022c443b4  Value=true  OutDataTypeStr=boolean
      settings: AttributesFormatString=%<OutDataTypeStr>
  Constant2 : Constant  RequirementInfo={} %GIDa_0e0c1627_bd48_4b73_8c17_b3e71d289e10  Value=GmOvrlStMgrLoaMtgtnStrtHaptcAmp
  Constant3 : Constant  RequirementInfo={} %GIDa_1283bd5f_c42e_4786_be01_cb33c6733a49  Value=GmOvrlStMgrLoaMtgtnHaptcFrq
  CopyRight2 : Subsystem  Description=|  mask(Copyright Information){none=on}
      | Copyright info block.                                               
      |                                                                     
      | Place copyright information at the top of every subsystem in design.
      mask prompts: none "No parameters"
      mask help: Place copyright information at the top of every subsystem in design.
      mask Display:
      | NxtrConf = 'Nexteer Confidential';
      | 
      | sys = bdroot; %handle for the current model ("system")
      | first = get_param(sys,'Created');
      | if(isempty(first))
      |     first = datestr(now,'yyyy');
      | else
      |     first = first(end-3:end);  %year is last four digits
      | end
      | 
      | last = get_param(sys,'LastModifiedDate');
      | if isempty(last)
      |     last = datestr(now,'yyyy');
      | else
      |     last = last(end-3:end);
      | end
      | 
      | if strcmp(first,last)
      |     fprintf('%s -- Copyright %s Nexteer',NxtrConf,first)
      | else
      |     fprintf('%s -- %s%s- %s Nexteer',NxtrConf,char(169),first,last)
      | end
  Data Store Read : DataStoreRead  DataStoreName=LoaMtgtnHaptcFbStrtOnRefTi
  GetTiSpan100MicroSec32bit : Subsystem
  If4 : If  IfExpression=u1  ShowElse=off
  Product1 : Product
  Relational Operator : RelationalOperator  OutDataTypeStr=boolean
  Set_True_LoaStAlreadyChk : Subsystem  TreatAsAtomicUnit=on
  HaptcFbEn : Outport
  HwOscnMotAmp : Outport  RequirementInfo={} %GIDa_da8b7ae1_79c3_4630_835c_267660e443df  Port=2
  HwOscnFrq : Outport  RequirementInfo={} %GIDa_fa4c2daf_88d1_442e_8c15_e617778cd142  Port=3
  wires:
  Constant/1 -> Product1/1
  Product1/1 -> Relational Operator/2
  Constant1/1 -> Product1/2
  If4/1 -> Set_True_LoaStAlreadyChk/Action
  Relational Operator/1 -> If4/1
  Data Store Read/1 -> GetTiSpan100MicroSec32bit/1(RefTmr)
  GetTiSpan100MicroSec32bit/1(TiSpan) -> Relational Operator/1
  Constant13/1 -> HaptcFbEn/1
  Constant3/1 -> HwOscnFrq/1
  Constant2/1 -> HwOscnMotAmp/1

== system CF009A_GmOvrlStMgr/GmOvrlStMgr/GmOvrlStMgrPer1/SysStOperate/Chk_LoaSt_IgnCntr_ AtStartUp/Set_True_LoaStAlreadyChk_HaptcFbOff ==
  Action Port : ActionPort  ActionType=else
  Constant : Constant  Value=0  OutDataTypeStr=single
  Constant1 : Constant  Value=HWOSCNFRQMIN_HZ_F32  OutDataTypeStr=single
  Constant2 : Constant  Value=true  OutDataTypeStr=boolean
      settings: AttributesFormatString=%<OutDataTypeStr>
  Constant9 : Constant  Value=false  OutDataTypeStr=boolean
      settings: AttributesFormatString=%<OutDataTypeStr>
  CopyRight2 : Subsystem  Description=|  mask(Copyright Information){none=on}
      | Copyright info block.                                               
      |                                                                     
      | Place copyright information at the top of every subsystem in design.
      mask prompts: none "No parameters"
      mask help: Place copyright information at the top of every subsystem in design.
      mask Display:
      | NxtrConf = 'Nexteer Confidential';
      | 
      | sys = bdroot; %handle for the current model ("system")
      | first = get_param(sys,'Created');
      | first = first(end-3:end);  %year is last four digits
      | 
      | last = get_param(sys,'LastModifiedDate');
      | if isempty(last)
      |     last = datestr(now,'yyyy');
      | else
      |     last = last(end-3:end);
      | end
      | 
      | if strcmp(first,last)
      |     fprintf('%s -- Copyright %s Nexteer',NxtrConf,first)
      | else
      |     fprintf('%s -- %s%s- %s Nexteer',NxtrConf,char(169),first,last)
      | end
  Data Store Write1 : DataStoreWrite  DataStoreName=LoaMtgtnHaptcFbStrtOnRefTi
  Data Store Write8 : DataStoreWrite  DataStoreName=LoaStChk
  GetRefTmr100MicroSec32bit : Subsystem
  HwOscnEna : Outport  RequirementInfo={} %GIDa_8b27570c_f12a_44bd_9f1b_a12f105bfe32
  HwOscnMotAmp : Outport  RequirementInfo={} %GIDa_9bc8c96c_d837_4e6b_9d2a_397928442c6b  Port=2
  HwOscnFrq : Outport  RequirementInfo={} %GIDa_14cb683a_9a4e_4ed2_8a6e_fb06c6026e0e  Port=3
  wires:
  GetRefTmr100MicroSec32bit/1(RefTmr) -> Data Store Write1/1
  Constant1/1 -> HwOscnFrq/1
  Constant/1 -> HwOscnMotAmp/1
  Constant9/1 -> HwOscnEna/1
  Constant2/1 -> Data Store Write8/1

== system CF009A_GmOvrlStMgr/GmOvrlStMgr/GmOvrlStMgrPer1/SysStOperate/Get_HaptcFb_After_StartUp/APAStAvl_AaptcStActv ==
  Action Port : ActionPort  ActionType=then
  Constant2 : Constant  RequirementInfo={} %GIDa_26ed30cd_65b7_497c_99c0_2c1cfdd65d5d  Value=GmOvrlStMgrHaptcAmp
  Constant3 : Constant  RequirementInfo={} %GIDa_3af3e024_021c_4d8b_9358_e76bd2cbdf8f  Value=GmOvrlStMgrHaptcFrq
  Constant9 : Constant  Value=true  OutDataTypeStr=boolean
      settings: AttributesFormatString=%<OutDataTypeStr>
  CopyRight2 : Subsystem  Description=|  mask(Copyright Information){none=on}
      | Copyright info block.                                               
      |                                                                     
      | Place copyright information at the top of every subsystem in design.
      mask prompts: none "No parameters"
      mask help: Place copyright information at the top of every subsystem in design.
      mask Display:
      | NxtrConf = 'Nexteer Confidential';
      | 
      | sys = bdroot; %handle for the current model ("system")
      | first = get_param(sys,'Created');
      | if(isempty(first))
      |     first = datestr(now,'yyyy');
      | else
      |     first = first(end-3:end);  %year is last four digits
      | end
      | 
      | last = get_param(sys,'LastModifiedDate');
      | if isempty(last)
      |     last = datestr(now,'yyyy');
      | else
      |     last = last(end-3:end);
      | end
      | 
      | if strcmp(first,last)
      |     fprintf('%s -- Copyright %s Nexteer',NxtrConf,first)
      | else
      |     fprintf('%s -- %s%s- %s Nexteer',NxtrConf,char(169),first,last)
      | end
  HwOscnEna : Outport  RequirementInfo={} %GIDa_47629f5c_8f25_4666_a146_71f8917c2095
  HwOscnMotAmp : Outport  RequirementInfo={} %GIDa_7d1b9b8e_a4d9_4512_9671_cecba50286e4  Port=2
  HwOscnFrq : Outport  RequirementInfo={} %GIDa_40ff6541_bf70_433b_bf6e_81869915c99d  Port=3
  wires:
  Constant3/1 -> HwOscnFrq/1
  Constant2/1 -> HwOscnMotAmp/1
  Constant9/1 -> HwOscnEna/1

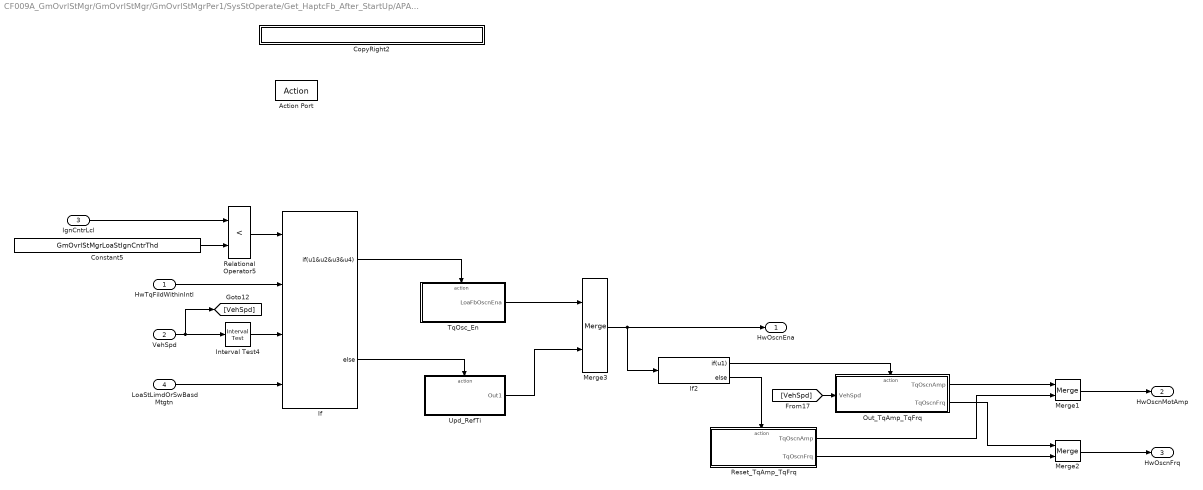
== system CF009A_GmOvrlStMgr/GmOvrlStMgr/GmOvrlStMgrPer1/SysStOperate/Get_HaptcFb_After_StartUp/APASt_NotAvl ==
  HwTqFildWithinIntl : Inport  RequirementInfo={} %GIDa_cc459f4f_ef8a_4d60_8375_9eec1001a331
  VehSpd : Inport  RequirementInfo={} %GIDa_7470b054_27ec_4b2a_a6ea_1766faf4dbc1  Port=2
  IgnCntrLcl : Inport  RequirementInfo={} %GIDa_7f00c7e6_1dc5_493c_83e8_51fe96291a10  Port=3
  LoaStLimdOrSwBasdMtgtn : Inport  RequirementInfo={} %GIDa_d7ddf5d2_779e_4bc0_a066_f8d511380f7a  Port=4
  Action Port : ActionPort  ActionType=elseif
  Constant5 : Constant  Value=GmOvrlStMgrLoaStIgnCntrThd
  CopyRight2 : Subsystem  Description=|  mask(Copyright Information){none=on}
      | Copyright info block.                                               
      |                                                                     
      | Place copyright information at the top of every subsystem in design.
      mask prompts: none "No parameters"
      mask help: Place copyright information at the top of every subsystem in design.
      mask Display:
      | NxtrConf = 'Nexteer Confidential';
      | 
      | sys = bdroot; %handle for the current model ("system")
      | first = get_param(sys,'Created');
      | if(isempty(first))
      |     first = datestr(now,'yyyy');
      | else
      |     first = first(end-3:end);  %year is last four digits
      | end
      | 
      | last = get_param(sys,'LastModifiedDate');
      | if isempty(last)
      |     last = datestr(now,'yyyy');
      | else
      |     last = last(end-3:end);
      | end
      | 
      | if strcmp(first,last)
      |     fprintf('%s -- Copyright %s Nexteer',NxtrConf,first)
      | else
      |     fprintf('%s -- %s%s- %s Nexteer',NxtrConf,char(169),first,last)
      | end
  If : If  NumInputs=4  IfExpression=u1&u2&u3&u4
  If2 : If  IfExpression=u1
  Interval Test4 : simulink/Logic and Bit Operations/Interval Test  IntervalClosedRight=on  uplimit=GmOvrlStMgrLoaMtgtnHaptcFbVehSpdMax  IntervalClosedLeft=on  lowlimit=GmOvrlStMgrLoaMtgtnHaptcFbVehSpdMin  OutDataTypeStr=boolean
  Merge1 : Merge
  Merge2 : Merge
  Merge3 : Merge
  Out_TqAmp_TqFrq : Subsystem  TreatAsAtomicUnit=on
  Relational Operator5 : RelationalOperator  Operator=<  OutDataTypeStr=boolean
  Reset_TqAmp_TqFrq : Subsystem  TreatAsAtomicUnit=on
  TqOsc_En : Subsystem  TreatAsAtomicUnit=on
  Upd_RefTi : Subsystem  TreatAsAtomicUnit=on
  HwOscnEna : Outport  RequirementInfo={} %GIDa_5788a13f_5bc7_4cac_a2cd_7377a94a3611
  HwOscnMotAmp : Outport  RequirementInfo={} %GIDa_f68b394c_8d0d_43c4_9707_2903078e112d  Port=2
  HwOscnFrq : Outport  RequirementInfo={} %GIDa_acfda0af_c439_4bb5_8d5a_b0d3cbfd6167  Port=3
  wires:
  Constant5/1 -> Relational Operator5/2
  HwTqFildWithinIntl/1 -> If/2
  VehSpd/1 -> [VehSpd], Interval Test4/1
  Relational Operator5/1 -> If/1
  IgnCntrLcl/1 -> Relational Operator5/1
  LoaStLimdOrSwBasdMtgtn/1 -> If/4
  If/1 -> TqOsc_En/Action
  If/2 -> Upd_RefTi/Action
  Merge3/1 -> If2/1, HwOscnEna/1
  If2/1 -> Out_TqAmp_TqFrq/Action
  If2/2 -> Reset_TqAmp_TqFrq/Action
  Reset_TqAmp_TqFrq/1(TqOscnAmp) -> Merge1/2
  Out_TqAmp_TqFrq/1(TqOscnAmp) -> Merge1/1
  Out_TqAmp_TqFrq/2(TqOscnFrq) -> Merge2/1
  Reset_TqAmp_TqFrq/2(TqOscnFrq) -> Merge2/2
  [VehSpd] -> Out_TqAmp_TqFrq/1(VehSpd)
  Merge1/1 -> HwOscnMotAmp/1
  Merge2/1 -> HwOscnFrq/1
  TqOsc_En/1(LoaFbOscnEna) -> Merge3/1
  Upd_RefTi/1(Out1) -> Merge3/2
  Interval Test4/1 -> If/3

== system CF009A_GmOvrlStMgr/GmOvrlStMgr/GmOvrlStMgrPer1/SysStOperate/Get_HaptcFb_After_StartUp/CopyRight2 ==

== system CF009A_GmOvrlStMgr/GmOvrlStMgr/GmOvrlStMgrPer1/SysStOperate/Get_HaptcFb_After_StartUp/else ==
  Action Port : ActionPort  ActionType=else
  Constant : Constant  Value=0  OutDataTypeStr=single
  Constant1 : Constant  Value=HWOSCNFRQMIN_HZ_F32  OutDataTypeStr=single
  Constant9 : Constant  Value=false  OutDataTypeStr=boolean
      settings: AttributesFormatString=%<OutDataTypeStr>
  CopyRight2 : Subsystem  Description=|  mask(Copyright Information){none=on}
      | Copyright info block.                                               
      |                                                                     
      | Place copyright information at the top of every subsystem in design.
      mask prompts: none "No parameters"
      mask help: Place copyright information at the top of every subsystem in design.
      mask Display:
      | NxtrConf = 'Nexteer Confidential';
      | 
      | sys = bdroot; %handle for the current model ("system")
      | first = get_param(sys,'Created');
      | if(isempty(first))
      |     first = datestr(now,'yyyy');
      | else
      |     first = first(end-3:end);  %year is last four digits
      | end
      | 
      | last = get_param(sys,'LastModifiedDate');
      | if isempty(last)
      |     last = datestr(now,'yyyy');
      | else
      |     last = last(end-3:end);
      | end
      | 
      | if strcmp(first,last)
      |     fprintf('%s -- Copyright %s Nexteer',NxtrConf,first)
      | else
      |     fprintf('%s -- %s%s- %s Nexteer',NxtrConf,char(169),first,last)
      | end
  HwOscnEna : Outport  RequirementInfo={} %GIDa_3280ee71_d8f3_4d09_a2fd_8ffc4630e987
  HwOscnMotAmp : Outport  RequirementInfo={} %GIDa_4d2b0a4a_9f58_449c_b512_e560f8e6ff6f  Port=2
  HwOscnFrq : Outport  RequirementInfo={} %GIDa_391d4338_8020_43b0_8a38_466840f22cda  Port=3
  wires:
  Constant1/1 -> HwOscnFrq/1
  Constant/1 -> HwOscnMotAmp/1
  Constant9/1 -> HwOscnEna/1

== system CF009A_GmOvrlStMgr/GmOvrlStMgr/GmOvrlStMgrPer1/Timer for HwHaptcEna/If Action Subsystem/CopyRight2 ==
